simulink model "chap3_10sim"  (Simulink 5.0)
settings: Solver=ode45  StartTime=0.0  StopTime=10  FixedStep=0.01  RelTol=1e-5
settings Model: LastModifiedBy=Administrator  ExtModeTrigMode=oneshot  ExtModeArmWhenConnect=off  LimitDataPoints=off  BooleanDataType=off

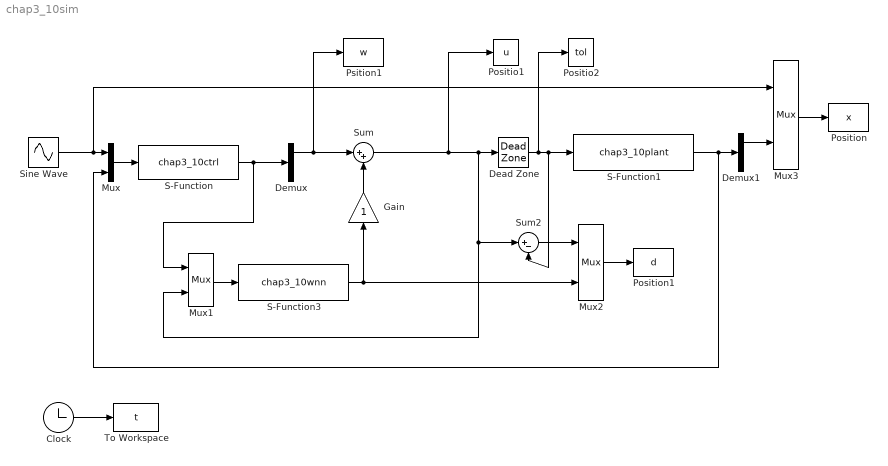
== system chap3_10sim ==
  Clock : Clock
      settings: Decimation=10
  Dead Zone : DeadZone  LowerValue=-5  UpperValue=5  SaturateOnIntegerOverflow=on
  Demux : Demux  Outputs=2
  Demux1 : Demux  Outputs=2
  Gain : Gain  Orientation=up  SaturateOnIntegerOverflow=on
  Mux{,1..3} (4 alike) : Mux  Inputs=2
  Positio1 : ToWorkspace  VariableName=u  SampleTime=-1  SaveFormat=Array
  Positio2 : ToWorkspace  VariableName=tol  SampleTime=-1  SaveFormat=Array
  Position : ToWorkspace  VariableName=x  SampleTime=-1  SaveFormat=Array
  Position1 : ToWorkspace  VariableName=d  SampleTime=-1  SaveFormat=Array
  Psition1 : ToWorkspace  VariableName=w  SampleTime=-1  SaveFormat=Array
  S-Function : S-Function  FunctionName=chap3_10ctrl
  S-Function1 : S-Function  FunctionName=chap3_10plant
  S-Function3 : S-Function  FunctionName=chap3_10wnn
  Sine Wave : Sin  Amplitude=0.5  Frequency=2  SampleTime=0
  Sum : Sum  Inputs=|++  SaturateOnIntegerOverflow=on
  Sum2 : Sum  Inputs=|+-  SaturateOnIntegerOverflow=on
  To Workspace : ToWorkspace  VariableName=t  SampleTime=-1  SaveFormat=Array
  wires:
  Sine Wave/1 -> Mux3/1, Mux/1
  Mux3/1 -> Position/1
  S-Function1/1 -> Mux/2, Demux1/1
  Mux/1 -> S-Function/1
  S-Function/1 -> Demux/1, Mux1/1
  Demux/1 -> Sum/1, Psition1/1
  Demux1/1 -> Mux3/2
  Dead Zone/1 -> Sum2/2, S-Function1/1, Positio2/1
  Sum/1 -> Dead Zone/1, Sum2/1, Mux1/2, Positio1/1
  Gain/1 -> Sum/2
  Mux1/1 -> S-Function3/1
  S-Function3/1 -> Gain/1, Mux2/2
  Mux2/1 -> Position1/1
  Sum2/1 -> Mux2/1
  Clock/1 -> To Workspace/1
